simulink model "xpccanisa"  (Simulink 4.00)
settings: Solver=FixedStepDiscrete  StartTime=0.0  StopTime=300  RelTol=1e-3
undefined symbols (not defined in the file or in its folder): bit, D4000, D7FFF, Standard
libraries: xpclib x5
settings Model: Creator=mvetsch  LastModifiedBy=mvetsch  RTWSystemTargetFile=xpctarget.tlc  RTWOptions="-aExtMode=1 -aForceParamTrailComments=0 -aInlineInvariantSignals=0 -aInlineParameters=0 -aLocalBlockOutputs=0 -aRL32IRQSourceModifier=\"Timer\" -aRL32LogBufSizeModifier=100000 -aRL32LogTETModifier=1 -aRL32ModeModifier=\"Real-Time\" -aRL32ObjectName=\"tg\" -aRL32ScopeModifier=1 -aRTWVerbose=1 -aRollThreshold=5 -aShowEliminatedStatements=1"  RTWTemplateMakefile=xpc_default_tmf  ExtModeMexFile=ext_xpc  ExtModeArmWhenConnect=off  OptimizeBlockIOStorage=off  BlockReductionOpt=off

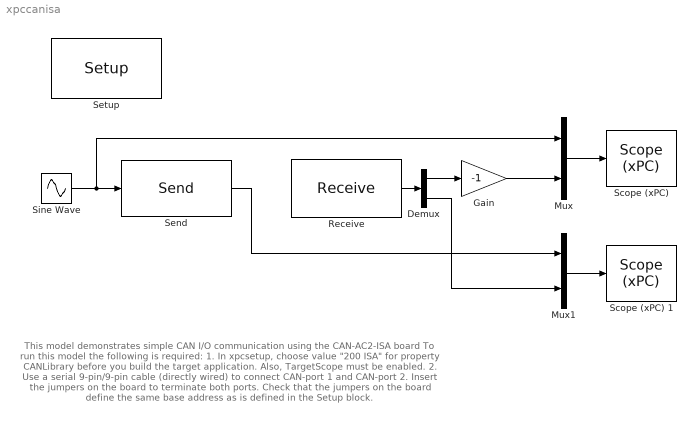
== system xpccanisa ==
  note: This model demonstrates simple CAN I/O communication using the CAN-AC2-ISA board
      |
      | To run this model the following is required:
      |
      | 1. In xpcsetup, choose value "200 ISA" for property CANLibrary before you build the
      | target application. Also, TargetScope must be enabled.
      |
      | 2. Use a serial 9-pin/9-pin cable (directly wired) to connect CAN-port 1 and CAN-port 2.
      | Insert the jumpers on the board to terminate both ports. Check that the jumpers on
      | the board define the same base address as is defined in the Setup block.
  Demux : Demux  Outputs=2  BusSelectionMode=off
  Gain : Gain  Gain=-1  Multiplication=Element-wise(K.*u)  SaturateOnIntegerOverflow=on
  Mux : Mux  Inputs=2
  Mux1 : Mux  Inputs=2
  "Receive " : xpclib/CAN/Softing/CAN-AC2-ISA Philips C200/Receive   board=1  canPort=CAN 2  range=Standard (11-bit)  ids=[50]  output=Data - Status  inten=off  ts=0.01  ididx=[0]
  "Scope (xPC) " : xpclib/Misc./Scope (xPC)   scopeno=1  scopetype=Target  viewmode=Graphical rolling  grid=on  ylimits=[0,0]  autostart=on  nosamples=250  noprepostsamples=0  interleave=1  triggermode=FreeRun  triggersignal=1  triggerlevel=0.0  triggerslope=either  triggerscope=1
  Scope (xPC) 1 : xpclib/Misc./Scope (xPC)   scopeno=2  scopetype=Target  viewmode=Numerical  grid=on  ylimits=[0,0]  autostart=on  nosamples=10  noprepostsamples=0  interleave=1  triggermode=FreeRun  triggersignal=1  triggerlevel=0.0  triggerslope=either  triggerscope=1
  "Send " : xpclib/CAN/Softing/CAN-AC2-ISA Philips C200/Send   board=1  canPort=CAN 1  range=Standard (11-bit)  ids=[50]  sizes=[8]  output=on  ts=0.01  ididx=[0]
  "Setup " : xpclib/CAN/Softing/CAN-AC2-ISA Philips C200/Setup   can1Baudrate=1 MBaud  can1UserBR=[1,1,4,3]  can2Baudrate=1 MBaud  can2UserBR=[1,1,4,3]  init=[]  term=[]  memBaseAddressL=2 (16k): D4000-D7FFF
  Sine Wave : Sin  Amplitude=1  Frequency=5  Phase=0  SampleTime=0.01
  wires:
  Sine Wave/1 -> "Send "/1, Mux/1
  "Receive "/1 -> Demux/1
  Demux/1 -> Gain/1
  Gain/1 -> Mux/2
  Mux/1 -> "Scope (xPC) "/1
  Mux1/1 -> Scope (xPC) 1/1
  "Send "/1 -> Mux1/1
  Demux/2 -> Mux1/2
